simulink model "Test"  (R2022a)
settings: Solver=VariableStepAuto  StartTime=0.0  StopTime=10  RelTol=1e-3
values from neighbouring files (symbols this model uses):
  kd_altitude = 0.475    [QuadcopterParameters.m]
  kd_attitude = 40    [QuadcopterParameters.m]
  KD_position = 0.85    [QuadcopterParameters.m]
  ki_altitude = 0.0275    [QuadcopterParameters.m]
  ki_attitude = 5    [QuadcopterParameters.m]
  KP_altitude = 0.15    [QuadcopterParameters.m]
  kp_attitude = 8.5    [QuadcopterParameters.m]
  KP_position = 0.175    [QuadcopterParameters.m]
  planeX = 30    [QuadcopterParameters.m]
  planeY = 30    [QuadcopterParameters.m]
  planeZ = 0.2    [QuadcopterParameters.m]
  propHoverSpeed = 600    [QuadcopterParameters.m]
  target = wayPoints(:,end)    [QuadcopterParameters.m]
  timeStamp = zeros(length(xWaypt),1)    [QuadcopterParameters.m]
  wayPoints = [xWaypt yWaypt zWaypt]'    [QuadcopterParameters.m]
  xrot = 0    [QuadcopterParameters.m]
  xStart = 0    [QuadcopterParameters.m]
  yrot = 0    [QuadcopterParameters.m]
  yStart = 0    [QuadcopterParameters.m]
  zrot = 0    [QuadcopterParameters.m]
  zStart = 0.06    [QuadcopterParameters.m]
undefined symbols (not defined in the file or in its folder): X, Y, Z
libraries: sm_lib x88, fl_lib x44, nesl_utility x37, slpidlib x4
(part 1 of 4)
settings Model: Creator=ADMIN  LastModifiedBy=ADMIN

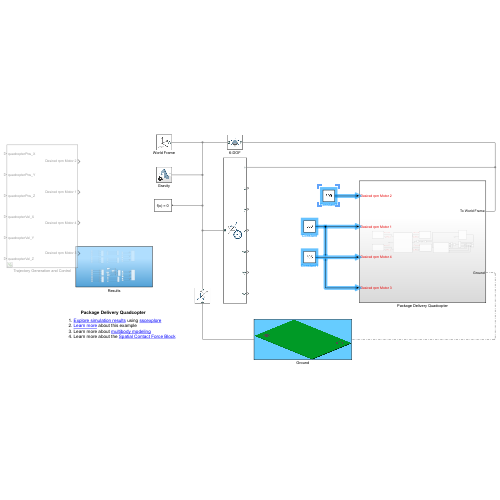
[thumbnail: Simulink's stored preview of the top-level diagram]
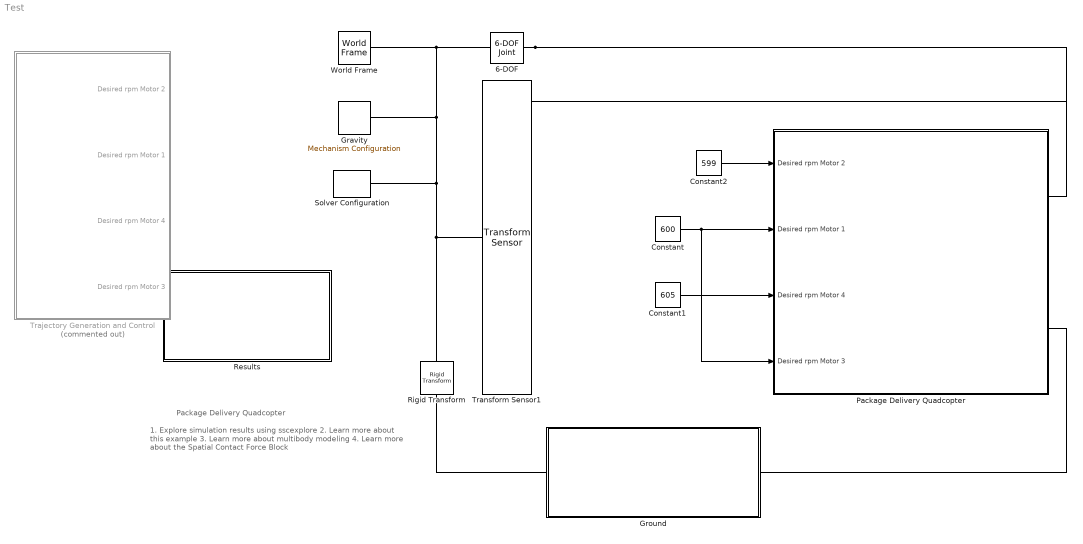
== system Test ==
  note: 1. Explore simulation results using sscexplore
      | 2. Learn more about this example
      | 3. Learn more about multibody modeling
      | 4. Learn more about the Spatial Contact Force Block
  note: Package Delivery Quadcopter
  6-DOF : sm_lib/Joints/6-DOF Joint  JointMode=Normal  SenseConstraintForce=off  SenseConstraintForceX=off  SenseConstraintForceY=off  SenseConstraintForceZ=off  SenseConstraintTorque=off  SenseConstraintTorqueX=off  SenseConstraintTorqueY=off  SenseConstraintTorqueZ=off  SenseTotalForce=off  SenseTotalForceX=off  SenseTotalForceY=off  SenseTotalForceZ=off  SenseTotalTorque=off  SenseTotalTorqueX=off  SenseTotalTorqueY=off  SenseTotalTorqueZ=off  CompositeWrenchDir=FollowerOnBase  CompositeWrenchFrame=BaseFrame  PxEquilibriumPosition=0  PxEquilibriumPositionUnits=m  PxSpringStiffness=0  PxSpringStiffnessUnits=N/m  PxDampingCoefficient=0  PxDampingCoefficientUnits=N/(m/s)  PxTorqueActuationMode=NoTorque  PxMotionActuationMode=ComputedMotion  PxSensePosition=off  PxSenseVelocity=off  PxSenseAcceleration=off  PxSenseTorqueForce=off  PxSenseLowerLimitTorqueForce=off  PxSenseUpperLimitTorqueForce=off  PxLowerLimitSpecify=off  PxLowerLimitBound=-1  PxLowerLimitBoundUnits=m  PxLowerLimitStiffness=1e6  PxLowerLimitStiffnessUnits=N/m  PxLowerLimitDamping=1e3  PxLowerLimitDampingUnits=N/(m/s)  PxLowerLimitTransitionRegionWidth=1e-4  PxLowerLimitTransitionRegionWidthUnits=m  PxUpperLimitSpecify=off  PxUpperLimitBound=1  PxUpperLimitBoundUnits=m  PxUpperLimitStiffness=1e6  PxUpperLimitStiffnessUnits=N/m  PxUpperLimitDamping=1e3  PxUpperLimitDampingUnits=N/(m/s)  PxUpperLimitTransitionRegionWidth=1e-4  PxUpperLimitTransitionRegionWidthUnits=m  PxPositionTargetSpecify=on  PxPositionTargetPriority=High  PxPositionTargetValue=xStart  PxPositionTargetValueUnits=m  PxVelocityTargetSpecify=off  PxVelocityTargetPriority=High  PxVelocityTargetValue=0  PxVelocityTargetValueUnits=m/s  PyEquilibriumPosition=0  PyEquilibriumPositionUnits=m  PySpringStiffness=0  PySpringStiffnessUnits=N/m  PyDampingCoefficient=0  PyDampingCoefficientUnits=N/(m/s)  PyTorqueActuationMode=NoTorque  PyMotionActuationMode=ComputedMotion  PySensePosition=off  PySenseVelocity=off  PySenseAcceleration=off  PySenseTorqueForce=off  PySenseLowerLimitTorqueForce=off  PySenseUpperLimitTorqueForce=off  PyLowerLimitSpecify=off  PyLowerLimitBound=-1  PyLowerLimitBoundUnits=m  PyLowerLimitStiffness=1e6  PyLowerLimitStiffnessUnits=N/m  PyLowerLimitDamping=1e3  PyLowerLimitDampingUnits=N/(m/s)  PyLowerLimitTransitionRegionWidth=1e-4  PyLowerLimitTransitionRegionWidthUnits=m  PyUpperLimitSpecify=off  PyUpperLimitBound=1  PyUpperLimitBoundUnits=m  PyUpperLimitStiffness=1e6  PyUpperLimitStiffnessUnits=N/m  PyUpperLimitDamping=1e3  PyUpperLimitDampingUnits=N/(m/s)  PyUpperLimitTransitionRegionWidth=1e-4  PyUpperLimitTransitionRegionWidthUnits=m  PyPositionTargetSpecify=on  PyPositionTargetPriority=High  PyPositionTargetValue=yStart  PyPositionTargetValueUnits=m  PyVelocityTargetSpecify=off  PyVelocityTargetPriority=High  PyVelocityTargetValue=0  PyVelocityTargetValueUnits=m/s  PzEquilibriumPosition=0  PzEquilibriumPositionUnits=m  PzSpringStiffness=0  PzSpringStiffnessUnits=N/m  PzDampingCoefficient=0  PzDampingCoefficientUnits=N/(m/s)  PzTorqueActuationMode=NoTorque  PzMotionActuationMode=ComputedMotion  PzSensePosition=off  PzSenseVelocity=off  PzSenseAcceleration=off  PzSenseTorqueForce=off  PzSenseLowerLimitTorqueForce=off  PzSenseUpperLimitTorqueForce=off  PzLowerLimitSpecify=off  PzLowerLimitBound=-1  PzLowerLimitBoundUnits=m  PzLowerLimitStiffness=1e6  PzLowerLimitStiffnessUnits=N/m  PzLowerLimitDamping=1e3  PzLowerLimitDampingUnits=N/(m/s)  PzLowerLimitTransitionRegionWidth=1e-4  PzLowerLimitTransitionRegionWidthUnits=m  PzUpperLimitSpecify=off  PzUpperLimitBound=1  PzUpperLimitBoundUnits=m  PzUpperLimitStiffness=1e6  PzUpperLimitStiffnessUnits=N/m  PzUpperLimitDamping=1e3  PzUpperLimitDampingUnits=N/(m/s)  PzUpperLimitTransitionRegionWidth=1e-4  PzUpperLimitTransitionRegionWidthUnits=m  PzPositionTargetSpecify=on  PzPositionTargetPriority=High  PzPositionTargetValue=zStart  PzPositionTargetValueUnits=m  PzVelocityTargetSpecify=off  PzVelocityTargetPriority=High  PzVelocityTargetValue=0  PzVelocityTargetValueUnits=m/s  SphDefPosRotationMethod=None  SphDefPosRotationAngleUnits=deg  SphDefPosRotationStandardAxis=+Z  SphDefPosRotationAngle=0.0  SphDefPosRotationArbitraryAxis=[0 0 1]  SphDefPosFollAlignAxisA=+X  SphDefPosBaseAlignAxisA=+Y  SphDefPosFollAlignAxisB=+Y  SphDefPosBaseAlignAxisB=+Z  SphDefPosRotationSequenceAxes=FollowerAxes  SphDefPosRotationSequence=XYX  SphDefPosRotationSequenceAngles=[0 0 0]  SphDefPosRotationSequenceAnglesUnits=deg  SphDefPosRotationMatrix=[1 0 0; 0 1 0; 0 0 1]  SphEqPosRotationMethod=None  SphEqPosRotationAngleUnits=deg  SphEqPosRotationStandardAxis=+Z  SphEqPosRotationAngle=0.0  SphEqPosRotationArbitraryAxis=[0 0 1]  SphEqPosFollAlignAxisA=+X  SphEqPosBaseAlignAxisA=+Y  SphEqPosFollAlignAxisB=+Y  SphEqPosBaseAlignAxisB=+Z  SphEqPosRotationSequenceAxes=FollowerAxes  SphEqPosRotationSequence=XYX  SphEqPosRotationSequenceAngles=[0 0 0]  SphEqPosRotationSequenceAnglesUnits=deg  SphEqPosRotationMatrix=[1 0 0; 0 1 0; 0 0 1]  SphSpringStiffness=0  SphSpringStiffnessUnits=N*m/deg  SphDampingCoefficient=0  SphDampingCoefficientUnits=N*m/(deg/s)  SphActuateTorqueX=off  SphActuateTorqueY=off  SphActuateTorqueZ=off  SphActuateTorque=off  SphTorqueActuationMode=NoTorque  SphMotionActuationMode=ComputedMotion  SphActuationFrame=BaseFrame  SphSensePosition=off  SphSenseVelocityX=off  SphSenseVelocityY=off  SphSenseVelocityZ=off  SphSenseVelocity=off  SphSenseAccelerationX=off  SphSenseAccelerationY=off  SphSenseAccelerationZ=off  SphSenseAcceleration=off  SphSenseTorqueX=off  SphSenseTorqueY=off  SphSenseTorqueZ=off  SphSenseTorqueForce=off  SphSenseLowerLimitTorqueMag=off  SphSenseUpperLimitTorqueMag=off  SphSensingFrame=BaseFrame  SphLowerLimitSpecify=off  SphLowerLimitBound=15  SphLowerLimitBoundUnits=deg  SphLowerLimitStiffness=1e4  SphLowerLimitStiffnessUnits=N*m/deg  SphLowerLimitDamping=10  SphLowerLimitDampingUnits=N*m/(deg/s)  SphLowerLimitTransitionRegionWidth=0.1  SphLowerLimitTransitionRegionWidthUnits=deg  SphUpperLimitSpecify=off  SphUpperLimitBound=45  SphUpperLimitBoundUnits=deg  SphUpperLimitStiffness=1e4  SphUpperLimitStiffnessUnits=N*m/deg  SphUpperLimitDamping=10  SphUpperLimitDampingUnits=N*m/(deg/s)  SphUpperLimitTransitionRegionWidth=0.1  SphUpperLimitTransitionRegionWidthUnits=deg  SphPositionTargetRotationMethod=RotationSequence  SphPositionTargetRotationAngleUnits=deg  SphPositionTargetRotationStandardAxis=+Y  SphPositionTargetRotationAngle=0  SphPositionTargetRotationArbitraryAxis=[0 0 1]  SphPositionTargetFollAlignAxisA=+X  SphPositionTargetBaseAlignAxisA=+Y  SphPositionTargetFollAlignAxisB=+Y  SphPositionTargetBaseAlignAxisB=+Z  SphPositionTargetRotationSequenceAxes=FollowerAxes  SphPositionTargetRotationSequence=XYZ  SphPositionTargetRotationSequenceAngles=[xrot yrot zrot]  SphPositionTargetRotationSequenceAnglesUnits=deg  SphPositionTargetRotationMatrix=[1 0 0; 0 1 0; 0 0 1]  SphPositionTargetSpecify=on  SphPositionTargetPriority=High  SphVelocityTargetValue=[0 0 0]  SphVelocityTargetValueUnits=deg/s  SphVelocityTargetSpecify=off  SphVelocityTargetPriority=High  SphVelocityTargetInFollowerFrame=on
  Constant : Constant  Value=600
  Constant1 : Constant  Value=605
  Constant2 : Constant  Value=599
  Gravity : sm_lib/Utilities/Mechanism Configuration  UniformGravity=Constant  GravityVector=[0 0 -9.80665]  GravityUnits=m/s^2  LinearizationDelta=0.001  JointModeTransitionNonlinearIterations=2
  Ground : Subsystem
      mask Display:
      | image(fullfile(matlabroot,'toolbox','physmod','sm','smdemos',...
      |     'quadcopter_package_delivery','images','ground.PNG'));
  Package Delivery Quadcopter : Subsystem
  "Results " : Subsystem
  Rigid Transform : sm_lib/Frames and Transforms/Rigid Transform  TranslationMethod=StandardAxis  TranslationStandardOffset=0.25  TranslationLengthUnit=m  TranslationStandardAxis=-Z  TranslationCartesianOffset=[0 0 0]  TranslationROffset=0  TranslationROffsetUnits=m  TranslationZOffset=0  TranslationZOffsetUnits=m  TranslationThetaOffset=0  TranslationThetaOffsetUnits=deg  RotationMethod=None  RotationAngleUnits=deg  RotationStandardAxis=+Z  RotationAngle=0.0  RotationArbitraryAxis=[0 0 1]  FollAlignAxisA=+X  BaseAlignAxisA=+Y  FollAlignAxisB=+Y  BaseAlignAxisB=+Z  RotationSequenceAxes=FollowerAxes  RotationSequence=XYX  RotationSequenceAngles=[0 0 0]  RotationSequenceAnglesUnits=deg  RotationMatrix=[1 0 0; 0 1 0; 0 0 1]
  Solver Configuration : nesl_utility/Solver Configuration  PhysicalDomain=network_engine_domain  SubClassName=solver  LeftPortType=input  RightPortType=generic  Tones=[]  Harmonics=[]  SimulateNoise=off  Profile=off  UseLocalSampling=off  EnableSwitchedLinearOptims=on  FrequencyDomain=off  UseCCode=off  RelTol=0.001  AbsTol=1e-06  MinStep=1e-09  ToWorkspace=off  RevertToSquareIcSolve=off  NumHomotopyIterations=100  PhasorMode=off  PhasorModeNumHarmonics=1  IndexReductionMethod=DerivativeReplacement  DoDC=off  ResidualTolerance=1e-09  UseLocalSolver=off  LocalSolverChoice=NE_BACKWARD_EULER_ADVANCER  LocalSolverSampleTime=Ts  DoFixedCost=off  MaxNonlinIter=3  MaxModeIter=2  ComputeImpulses=off  ImpulseIterations=2  LinearAlgebra=auto  LinearAlgebraNumThread=0  EquationFormulation=NE_TIME_EF  DelaysMemoryBudget=1024  AutomaticFiltering=on  FilteringTimeConstant=0.001  PartitionStorageMethod=AS_NEEDED  PartitionMemoryBudget=1024  PartitionMethod=ROBUST
      settings: SourceProductBaseCode=SS,PW,VE
  Trajectory Generation and Control : Subsystem  Commented=on
  Transform Sensor1 : sm_lib/Frames and Transforms/Transform Sensor  MeasurementFrame=NonRotatingBase  SenseAngle=off  SenseAxis=off  SenseAngle1=off  SenseAngle2=off  SenseAngle3=off  SenseQ=off  SenseR=off  SenseOmegaX=off  SenseOmegaY=off  SenseOmegaZ=off  SenseOmega1=off  SenseOmega2=off  SenseOmega3=off  SenseQDot=off  SenseRDot=off  SenseAlphaX=off  SenseAlphaY=off  SenseAlphaZ=off  SenseAlpha1=off  SenseAlpha2=off  SenseAlpha3=off  SenseQDDot=off  SenseRDDot=off  SenseX=on  SenseY=on  SenseZ=on  SenseRad=off  SenseAzim=off  SenseDist=off  SenseInc=off  SenseXDot=on  SenseYDot=on  SenseZDot=on  SenseRadDot=off  SenseAzimDot=off  SenseDistDot=off  SenseIncDot=off  SenseXDDot=off  SenseYDDot=off  SenseZDDot=off  SenseRadDDot=off  SenseAzimDDot=off  SenseDistDDot=off  SenseIncDDot=off
  World Frame : sm_lib/Frames and Transforms/World Frame
  wires:
  Constant2/1 -> Package Delivery Quadcopter/1(Desired rpm Motor 2)
  Constant1/1 -> Package Delivery Quadcopter/3(Desired rpm Motor 4)
  Constant/1 -> Package Delivery Quadcopter/4(Desired rpm Motor 3), Package Delivery Quadcopter/2("Desired rpm Motor 1 ")
  connections:
  Rigid Transform/LConn1 -- Transform Sensor1/LConn1 -- Gravity/RConn1 -- 6-DOF/LConn1 -- World Frame/RConn1 -- Solver Configuration/RConn1
  6-DOF/RConn1 -- Transform Sensor1/RConn1 -- Package Delivery Quadcopter/RConn1
  Package Delivery Quadcopter/RConn2 -- Ground/LConn1
  Rigid Transform/RConn1 -- Ground/RConn1

== system Test/Ground ==
  Ground : sm_lib/Body Elements/Brick Solid  GraphicAmbientColor=[0.15 0.15 0.15 1.0]  BasedOnType=Density  BrickDimensions=[planeX planeY planeZ]  BrickDimensionUnits=m  CenterOfMass=[0 0 0]  CenterOfMassUnits=m  GraphicDiffuseColor=[0.0 0.8 0.2]  Density=1000  DensityUnits=kg/m^3  DoExposeReferenceFrame=on  GraphicEmissiveColor=[0.0 0.0 0.0 1.0]  ExportEntireGeometry=on  SerializedFrames=<Frames><Frame><Id>Frame1</Id><Value><Name>Lp</Name><Origin><Source>GeometricFeature</Source><FeatureName>+z surface</FeatureName></Origin><PrimaryAxis><DefinedDirection>+Z</DefinedDirection><Source>ReferenceFrame</Source><SourceDirection>+Z</SourceDirection><FeatureName></FeatureName></PrimaryAxis><SecondaryAxis><DefinedDirection>+X</DefinedDirection><Source>ReferenceFrame</Source><SourceDirection>+X</SourceDirection><FeatureName></FeatureName></SecondaryAxis></Value></Frame></Frames>  MarkerShape=Sphere  MarkerSize=10  GraphicType=FromGeometry  InertiaType=CalculateFromGeometry  Mass=1  MassUnits=kg  MomentsOfInertia=[1 1 1]  MomentsOfInertiaUnits=kg*m^2  GraphicOpacity=1  ProductsOfInertia=[0 0 0]  ProductsOfInertiaUnits=kg*m^2  GraphicShininess=75  GraphicSpecularColor=[0.5 0.5 0.5 1.0]  GraphicVisPropType=SimpleVisualProperties
  Launchpad : sm_lib/Body Elements/Extruded Solid  GraphicAmbientColor=[0.15 0.15 0.15 1.0]  BasedOnType=Density  CenterOfMass=[0 0 0]  CenterOfMassUnits=m  GraphicDiffuseColor=[0.4 0.4 0.4]  ExportConvexHullGeometry=off  ExtrusionCrossSection=[0.15 0.15; -0.15 0.15; -0.15 0.75; -0.6 0.75; -0.6 -0.75; -0.15 -0.75; -0.15 -0.15; 0.15 -0.15; 0.15 -0.75; 0.6 -0.75; 0.6 0.75; 0.15 0.75]*0.25  ExtrusionCrossSectionUnits=m  Density=1  DensityUnits=kg/m^3  DoExposeReferenceFrame=on  GraphicEmissiveColor=[0.0 0.0 0.0 1.0]  ExportEntireGeometry=off  ExtrusionLength=0.002  ExtrusionLengthUnits=m  ExtrusionType=General  SerializedFrames=<Frames/>  MarkerShape=Sphere  MarkerSize=10  GraphicType=FromGeometry  InertiaType=CalculateFromGeometry  Mass=1  MassUnits=kg  MomentsOfInertia=[1 1 1]  MomentsOfInertiaUnits=kg*m^2  PolygonNumSides=3  GraphicOpacity=1.0  PolygonOuterRadius=1  PolygonOuterRadiusUnits=m  ProductsOfInertia=[0 0 0]  ProductsOfInertiaUnits=kg*m^2  GraphicShininess=75  GraphicSpecularColor=[0.5 0.5 0.5 1.0]  GraphicVisPropType=SimpleVisualProperties
  Revolved Solid : sm_lib/Body Elements/Revolved Solid  GraphicAmbientColor=[0.15 0.15 0.15 1.0]  BasedOnType=Density  CenterOfMass=[0 0 0]  CenterOfMassUnits=m  GraphicDiffuseColor=[0.4 0.4 0.4]  ExportConvexHullGeometry=off  Density=1000  DensityUnits=kg/m^3  DoExposeReferenceFrame=on  GraphicEmissiveColor=[0.0 0.0 0.0 1.0]  ExportEntireGeometry=off  SerializedFrames=<Frames/>  MarkerShape=Sphere  MarkerSize=10  GraphicType=FromGeometry  InertiaType=CalculateFromGeometry  Mass=1  MassUnits=kg  MomentsOfInertia=[1 1 1]  MomentsOfInertiaUnits=kg*m^2  GraphicOpacity=1.0  ProductsOfInertia=[0 0 0]  ProductsOfInertiaUnits=kg*m^2  RevolutionCrossSection=[0.5 0.001; 0.5 -0.001; 0.75 -0.001; 0.75 0.001]*0.65  RevolutionCrossSectionUnits=m  RevolutionAngle=180  RevolutionAngleUnits=deg  RevolutionExtent=Full  GraphicShininess=75  GraphicSpecularColor=[0.5 0.5 0.5 1.0]  GraphicVisPropType=SimpleVisualProperties
  Rigid Transform1 : sm_lib/Frames and Transforms/Rigid Transform  TranslationMethod=Cartesian  TranslationStandardOffset=0  TranslationLengthUnit=m  TranslationStandardAxis=+Z  TranslationCartesianOffset=[xStart yStart 0 ]  TranslationROffset=0  TranslationROffsetUnits=m  TranslationZOffset=0  TranslationZOffsetUnits=m  TranslationThetaOffset=0  TranslationThetaOffsetUnits=deg  RotationMethod=None  RotationAngleUnits=deg  RotationStandardAxis=+Z  RotationAngle=0.0  RotationArbitraryAxis=[0 0 1]  FollAlignAxisA=+X  BaseAlignAxisA=+Y  FollAlignAxisB=+Y  BaseAlignAxisB=+Z  RotationSequenceAxes=FollowerAxes  RotationSequence=XYX  RotationSequenceAngles=[0 0 0]  RotationSequenceAnglesUnits=deg  RotationMatrix=[1 0 0; 0 1 0; 0 0 1]
  Rigid Transform12 : sm_lib/Frames and Transforms/Rigid Transform  TranslationMethod=Cartesian  TranslationStandardOffset=0  TranslationLengthUnit=m  TranslationStandardAxis=+Z  TranslationCartesianOffset=[target(1) target(2) 0 ]  TranslationROffset=0  TranslationROffsetUnits=m  TranslationZOffset=0  TranslationZOffsetUnits=m  TranslationThetaOffset=0  TranslationThetaOffsetUnits=deg  RotationMethod=None  RotationAngleUnits=deg  RotationStandardAxis=+Z  RotationAngle=0.0  RotationArbitraryAxis=[0 0 1]  FollAlignAxisA=+X  BaseAlignAxisA=+Y  FollAlignAxisB=+Y  BaseAlignAxisB=+Z  RotationSequenceAxes=FollowerAxes  RotationSequence=XYX  RotationSequenceAngles=[0 0 0]  RotationSequenceAnglesUnits=deg  RotationMatrix=[1 0 0; 0 1 0; 0 0 1]
  Target Marker : sm_lib/Body Elements/Revolved Solid  GraphicAmbientColor=[0.15 0.15 0.15 1.0]  BasedOnType=Density  CenterOfMass=[0 0 0]  CenterOfMassUnits=m  GraphicDiffuseColor=[0.4 0.4 0.4]  ExportConvexHullGeometry=off  Density=1000  DensityUnits=kg/m^3  DoExposeReferenceFrame=on  GraphicEmissiveColor=[0.0 0.0 0.0 1.0]  ExportEntireGeometry=off  SerializedFrames=<Frames/>  MarkerShape=Sphere  MarkerSize=10  GraphicType=FromGeometry  InertiaType=CalculateFromGeometry  Mass=1  MassUnits=kg  MomentsOfInertia=[1 1 1]  MomentsOfInertiaUnits=kg*m^2  GraphicOpacity=1.0  ProductsOfInertia=[0 0 0]  ProductsOfInertiaUnits=kg*m^2  RevolutionCrossSection=[0.5 0.001; 0.5 -0.001; 0.75 -0.001; 0.75 0.001]*0.75  RevolutionCrossSectionUnits=m  RevolutionAngle=180  RevolutionAngleUnits=deg  RevolutionExtent=Full  GraphicShininess=75  GraphicSpecularColor=[0.5 0.5 0.5 1.0]  GraphicVisPropType=SimpleVisualProperties
  Package : PMIOPort  Side=Left
  World Frame : PMIOPort  Port=2  Side=Right
  connections:
  Package/RConn1 -- Ground/LConn2
  Rigid Transform12/RConn1 -- Target Marker/RConn1
  Rigid Transform12/LConn1 -- Rigid Transform1/LConn1 -- Ground/LConn1
  Launchpad/RConn1 -- Revolved Solid/RConn1 -- Rigid Transform1/RConn1
  World Frame/RConn1 -- Ground/RConn1

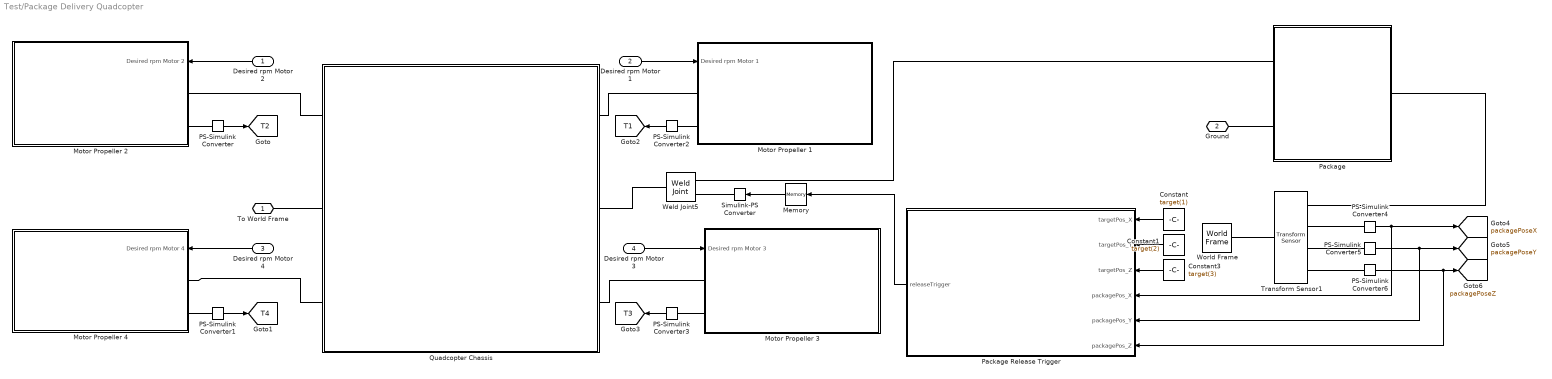
== system Test/Package Delivery Quadcopter ==
  Desired rpm Motor 2 : Inport
  "Desired rpm Motor 1 " : Inport  Port=2
  Desired rpm Motor 4 : Inport  Port=3
  Desired rpm Motor 3 : Inport  Port=4
  Constant : Constant  Value=target(1)
  Constant1 : Constant  Value=target(2)
  Constant3 : Constant  Value=target(3)
  Memory : Memory
  Motor Propeller 1 : Subsystem
  Motor Propeller 2 : Subsystem
      mask Display:
      | image(fullfile(matlabroot,'toolbox','physmod','sm','smdemos',...
      |     'quadcopter_package_delivery','images','propeller2.PNG'));
  "Motor Propeller 3 " : Subsystem
      mask Display:
      | image(fullfile(matlabroot,'toolbox','physmod','sm','smdemos',...
      |     'quadcopter_package_delivery','images','propeller3.PNG'));
  Motor Propeller 4 : Subsystem
      mask Display:
      | image(fullfile(matlabroot,'toolbox','physmod','sm','smdemos',...
      |     'quadcopter_package_delivery','images','propeller4.PNG'));
  PS-Simulink Converter{,1..6} (7 alike) : nesl_utility/PS-Simulink Converter  PhysicalDomain=network_engine_domain  SubClassName=ps_output  LeftPortType=input  RightPortType=output  PseudoPeriodic=off  Frequencies=[]  VectorFormat=1-D array  Unit=inherit  AffineConversion=off
      settings: SourceProductBaseCode=SS,PW,VE
  Package : Subsystem
      mask Display:
      | image(fullfile(matlabroot,'toolbox','physmod','sm','smdemos',...
      |     'quadcopter_package_delivery','images','medical_kit.png'));
  Package Release Trigger : MATLAB Function  TreatAsAtomicUnit=on
  Quadcopter Chassis : Subsystem
  Simulink-PS Converter : nesl_utility/Simulink-PS Converter  PhysicalDomain=network_engine_domain  SubClassName=ps_input  LeftPortType=input  RightPortType=output  PseudoPeriodic=off  Frequencies=[]  NoiseDistribution=none  NoiseParameters=[]  Unit=1  AffineConversion=off  FilteringAndDerivatives=provide  SimscapeFilterOrder=1  InputFilterTimeConstant=0.001  UdotUserProvided=0
      settings: SourceProductBaseCode=SS,PW,VE
  Transform Sensor1 : sm_lib/Frames and Transforms/Transform Sensor  MeasurementFrame=World  SenseAngle=off  SenseAxis=off  SenseAngle1=off  SenseAngle2=off  SenseAngle3=off  SenseQ=off  SenseR=off  SenseOmegaX=off  SenseOmegaY=off  SenseOmegaZ=off  SenseOmega1=off  SenseOmega2=off  SenseOmega3=off  SenseQDot=off  SenseRDot=off  SenseAlphaX=off  SenseAlphaY=off  SenseAlphaZ=off  SenseAlpha1=off  SenseAlpha2=off  SenseAlpha3=off  SenseQDDot=off  SenseRDDot=off  SenseX=on  SenseY=on  SenseZ=on  SenseRad=off  SenseAzim=off  SenseDist=off  SenseInc=off  SenseXDot=off  SenseYDot=off  SenseZDot=off  SenseRadDot=off  SenseAzimDot=off  SenseDistDot=off  SenseIncDot=off  SenseXDDot=off  SenseYDDot=off  SenseZDDot=off  SenseRadDDot=off  SenseAzimDDot=off  SenseDistDDot=off  SenseIncDDot=off
  Weld Joint5 : sm_lib/Joints/Weld Joint  JointMode=ProvidedByInput  SenseConstraintForce=off  SenseConstraintForceX=off  SenseConstraintForceY=off  SenseConstraintForceZ=off  SenseConstraintTorque=off  SenseConstraintTorqueX=off  SenseConstraintTorqueY=off  SenseConstraintTorqueZ=off  SenseTotalForce=off  SenseTotalForceX=off  SenseTotalForceY=off  SenseTotalForceZ=off  SenseTotalTorque=off  SenseTotalTorqueX=off  SenseTotalTorqueY=off  SenseTotalTorqueZ=off  CompositeWrenchDir=FollowerOnBase  CompositeWrenchFrame=BaseFrame
  World Frame : sm_lib/Frames and Transforms/World Frame
  To World Frame : PMIOPort  Side=Right
  Ground : PMIOPort  Port=2  Side=Right
  tag scope: T1=global, T2=global, T3=global, T4=global, packagePoseX=global, packagePoseY=global, packagePoseZ=global
  wires:
  PS-Simulink Converter/1 -> [T2]
  PS-Simulink Converter1/1 -> [T4]
  PS-Simulink Converter2/1 -> [T1]
  PS-Simulink Converter3/1 -> [T3]
  Desired rpm Motor 2/1 -> Motor Propeller 2/1(Desired rpm Motor 2)
  "Desired rpm Motor 1 "/1 -> Motor Propeller 1/1(Desired rpm Motor 1)
  Desired rpm Motor 4/1 -> Motor Propeller 4/1(Desired rpm Motor 4)
  Desired rpm Motor 3/1 -> "Motor Propeller 3 "/1(Desired rpm Motor 3)
  Memory/1 -> Simulink-PS Converter/1
  PS-Simulink Converter4/1 -> Package Release Trigger/4(packagePos_X), [packagePoseX]
  PS-Simulink Converter6/1 -> Package Release Trigger/6(packagePos_Z), [packagePoseZ]
  Package Release Trigger/1(releaseTrigger) -> Memory/1
  PS-Simulink Converter5/1 -> Package Release Trigger/5(packagePos_Y), [packagePoseY]
  Constant/1 -> Package Release Trigger/1(targetPos_X)
  Constant1/1 -> Package Release Trigger/2(targetPos_Y)
  Constant3/1 -> Package Release Trigger/3(targetPos_Z)
  connections:
  Motor Propeller 2/LConn1 -- Quadcopter Chassis/LConn1
  Motor Propeller 1/LConn1 -- Quadcopter Chassis/RConn1
  PS-Simulink Converter/LConn1 -- Motor Propeller 2/LConn2
  PS-Simulink Converter1/LConn1 -- Motor Propeller 4/LConn2
  PS-Simulink Converter2/LConn1 -- Motor Propeller 1/LConn2
  PS-Simulink Converter3/LConn1 -- "Motor Propeller 3 "/LConn2
  "Motor Propeller 3 "/LConn1 -- Quadcopter Chassis/RConn3
  Transform Sensor1/RConn1 -- Package/RConn1
  Ground/RConn1 -- Package/LConn2
  Transform Sensor1/RConn4 -- PS-Simulink Converter6/LConn1
  Transform Sensor1/RConn2 -- PS-Simulink Converter4/LConn1
  Transform Sensor1/RConn3 -- PS-Simulink Converter5/LConn1
  Simulink-PS Converter/RConn1 -- Weld Joint5/LConn2
  Package/LConn1 -- Weld Joint5/LConn1
  World Frame/RConn1 -- Transform Sensor1/LConn1
  Motor Propeller 4/LConn1 -- Quadcopter Chassis/LConn3
  To World Frame/RConn1 -- Quadcopter Chassis/LConn2
  Quadcopter Chassis/RConn2 -- Weld Joint5/RConn1

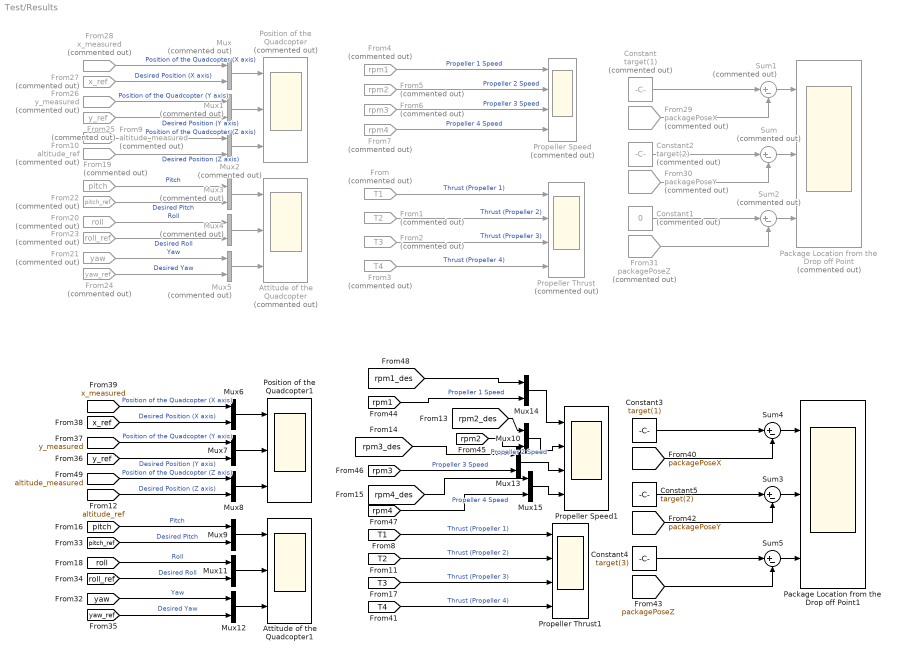
== system Test/Results  ==
  Attitude of the Quadcopter : Scope  Commented=on  NumInputPorts=3
  Attitude of the Quadcopter1 : Scope  NumInputPorts=3
  Constant : Constant  Commented=on  Value=target(1)
  Constant1 : Constant  Commented=on  Value=0
  Constant2 : Constant  Commented=on  Value=target(2)
  Constant3 : Constant  Value=target(1)
  Constant4 : Constant  Value=target(3)
  Constant5 : Constant  Value=target(2)
  From : From  Commented=on  GotoTag=T1  TagVisibility=global
  From1 : From  Commented=on  GotoTag=T2  TagVisibility=global
  From10 : From  Commented=on  GotoTag=altitude_ref  TagVisibility=global
  From19 : From  Commented=on  GotoTag=pitch  TagVisibility=global
  From2 : From  Commented=on  GotoTag=T3  TagVisibility=global
  From20 : From  Commented=on  GotoTag=roll  TagVisibility=global
  From21 : From  Commented=on  GotoTag=yaw  TagVisibility=global
  From22 : From  Commented=on  GotoTag=pitch_ref  TagVisibility=global
  From23 : From  Commented=on  GotoTag=roll_ref  TagVisibility=global
  From24 : From  Commented=on  GotoTag=yaw_ref  TagVisibility=global
  From25 : From  Commented=on  GotoTag=y_ref  TagVisibility=global
  From26 : From  Commented=on  GotoTag=y_measured  TagVisibility=global
  From27 : From  Commented=on  GotoTag=x_ref  TagVisibility=global
  From28 : From  Commented=on  GotoTag=x_measured  TagVisibility=global
  From29 : From  Commented=on  GotoTag=packagePoseX  TagVisibility=global
  From3 : From  Commented=on  GotoTag=T4  TagVisibility=global
  From30 : From  Commented=on  GotoTag=packagePoseY  TagVisibility=global
  From31 : From  Commented=on  GotoTag=packagePoseZ  TagVisibility=global
  From4 : From  Commented=on  GotoTag=rpm1  TagVisibility=global
  From5 : From  Commented=on  GotoTag=rpm2  TagVisibility=global
  From6 : From  Commented=on  GotoTag=rpm3  TagVisibility=global
  From7 : From  Commented=on  GotoTag=rpm4  TagVisibility=global
  From9 : From  Commented=on  GotoTag=altitude_measured  TagVisibility=global
  Mux{,1..5} (6 alike) : Mux  Commented=on  Inputs=2
  Mux{6..15} (10 alike) : Mux  Inputs=2
  Package Location from the Drop off Point : Scope  Commented=on  NumInputPorts=3
  Package Location from the Drop off Point1 : Scope  NumInputPorts=3
  Position of the Quadcopter : Scope  Commented=on  NumInputPorts=3
  Position of the Quadcopter1 : Scope  NumInputPorts=3
  Propeller Speed : Scope  Commented=on  NumInputPorts=4
  Propeller Speed1 : Scope  NumInputPorts=4
  Propeller Thrust : Scope  Commented=on  NumInputPorts=4
  Propeller Thrust1 : Scope  NumInputPorts=4
  Sum : Sum  Commented=on  Inputs=|+-
  Sum1 : Sum  Commented=on  Inputs=|+-
  Sum2 : Sum  Commented=on  Inputs=|+-
  Sum3 : Sum  Inputs=|+-
  Sum4 : Sum  Inputs=|+-
  Sum5 : Sum  Inputs=|+-
  wires:
  From4/1 -> Propeller Speed/1  "Propeller 1 Speed"
  From5/1 -> Propeller Speed/2  "Propeller 2 Speed"
  From6/1 -> Propeller Speed/3  "Propeller 3 Speed"
  From7/1 -> Propeller Speed/4  "Propeller 4 Speed"
  From10/1 -> Mux2/2  "Desired Position (Z axis)"
  From9/1 -> Mux2/1  "Position of the Quadcopter (Z axis)"
  From19/1 -> Mux3/1  "Pitch"
  From20/1 -> Mux4/1  "Roll"
  From21/1 -> Mux5/1  "Yaw"
  From22/1 -> Mux3/2  "Desired Pitch"
  From23/1 -> Mux4/2  "Desired Roll"
  From24/1 -> Mux5/2  "Desired Yaw"
  From25/1 -> Mux1/2  "Desired Position (Y axis)"
  From26/1 -> Mux1/1  "Position of the Quadcopter (Y axis)"
  From27/1 -> Mux/2  "Desired Position (X axis)"
  From28/1 -> Mux/1  "Position of the Quadcopter (X axis)"
  From31/1 -> Sum2/2
  Constant1/1 -> Sum2/1
  Constant2/1 -> Sum/1
  From30/1 -> Sum/2
  Constant/1 -> Sum1/1
  From29/1 -> Sum1/2
  Sum/1 -> Package Location from the Drop off Point/2
  Sum2/1 -> Package Location from the Drop off Point/3
  Mux1/1 -> Position of the Quadcopter/2
  Mux/1 -> Position of the Quadcopter/1
  Mux2/1 -> Position of the Quadcopter/3
  Mux4/1 -> Attitude of the Quadcopter/2
  Mux3/1 -> Attitude of the Quadcopter/1
  Mux5/1 -> Attitude of the Quadcopter/3
  From2/1 -> Propeller Thrust/3  "Thrust (Propeller 3)"
  From1/1 -> Propeller Thrust/2  "Thrust (Propeller 2)"
  From/1 -> Propeller Thrust/1  "Thrust (Propeller 1)"
  From3/1 -> Propeller Thrust/4  "Thrust (Propeller 4)"
  Sum1/1 -> Package Location from the Drop off Point/1
  [rpm3_des] -> Mux13/1
  [rpm3] -> Mux13/2  "Propeller 3 Speed"
  Mux15/1 -> Propeller Speed1/4
  Mux6/1 -> Position of the Quadcopter1/1
  [T3] -> Propeller Thrust1/3  "Thrust (Propeller 3)"
  Mux10/1 -> Propeller Speed1/2
  Sum4/1 -> Package Location from the Drop off Point1/1
  [T4] -> Propeller Thrust1/4  "Thrust (Propeller 4)"
  Mux12/1 -> Attitude of the Quadcopter1/3
  [pitch_ref] -> Mux9/2  "Desired Pitch"
  Constant3/1 -> Sum4/1
  [yaw] -> Mux12/1  "Yaw"
  [x_ref] -> Mux6/2  "Desired Position (X axis)"
  [rpm2] -> Mux10/2  "Propeller 2 Speed"
  [T2] -> Propeller Thrust1/2  "Thrust (Propeller 2)"
  [x_measured] -> Mux6/1  "Position of the Quadcopter (X axis)"
  Mux9/1 -> Attitude of the Quadcopter1/1
  Mux11/1 -> Attitude of the Quadcopter1/2
  [altitude_ref] -> Mux8/2  "Desired Position (Z axis)"
  Constant5/1 -> Sum3/1
  Sum3/1 -> Package Location from the Drop off Point1/2
  [y_ref] -> Mux7/2  "Desired Position (Y axis)"
  [roll] -> Mux11/1  "Roll"
  [rpm1] -> Mux14/2  "Propeller 1 Speed"
  [y_measured] -> Mux7/1  "Position of the Quadcopter (Y axis)"
  [packagePoseX] -> Sum4/2
  Constant4/1 -> Sum5/1
  [rpm2_des] -> Mux10/1
  [packagePoseZ] -> Sum5/2
  Mux13/1 -> Propeller Speed1/3
  [rpm4] -> Mux15/2  "Propeller 4 Speed"
  [yaw_ref] -> Mux12/2  "Desired Yaw"
  Sum5/1 -> Package Location from the Drop off Point1/3
  [packagePoseY] -> Sum3/2
  Mux14/1 -> Propeller Speed1/1
  [roll_ref] -> Mux11/2  "Desired Roll"
  Mux7/1 -> Position of the Quadcopter1/2
  [rpm1_des] -> Mux14/1
  Mux8/1 -> Position of the Quadcopter1/3
  [pitch] -> Mux9/1  "Pitch"
  [T1] -> Propeller Thrust1/1  "Thrust (Propeller 1)"
  [rpm4_des] -> Mux15/1
  [altitude_measured] -> Mux8/1  "Position of the Quadcopter (Z axis)"

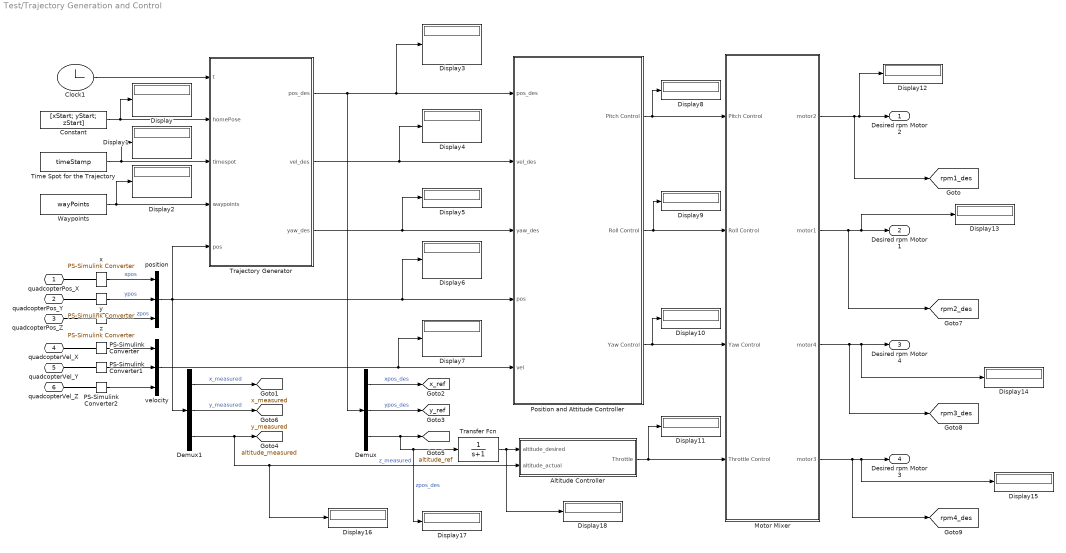
== system Test/Trajectory Generation and Control ==
  Altitude Controller : Subsystem
  Clock1 : Clock
  Constant : Constant  Value=[xStart; yStart; zStart]
  Demux : Demux  Outputs=3
  Demux1 : Demux  Outputs=3
  Display{,1..18} (19 alike) : Display
  Motor Mixer : Subsystem
  PS-Simulink Converter : nesl_utility/PS-Simulink Converter  PhysicalDomain=network_engine_domain  SubClassName=ps_output  LeftPortType=input  RightPortType=output  PseudoPeriodic=off  Frequencies=[]  VectorFormat=1-D array  Unit=inherit  AffineConversion=off
      settings: SourceProductBaseCode=SS,PW,VE
  PS-Simulink Converter1 : nesl_utility/PS-Simulink Converter  PhysicalDomain=network_engine_domain  SubClassName=ps_output  LeftPortType=input  RightPortType=output  PseudoPeriodic=off  Frequencies=[]  VectorFormat=1-D array  Unit=inherit  AffineConversion=off
      settings: SourceProductBaseCode=SS,PW,VE
  PS-Simulink Converter2 : nesl_utility/PS-Simulink Converter  PhysicalDomain=network_engine_domain  SubClassName=ps_output  LeftPortType=input  RightPortType=output  PseudoPeriodic=off  Frequencies=[]  VectorFormat=1-D array  Unit=inherit  AffineConversion=off
      settings: SourceProductBaseCode=SS,PW,VE
  Position and Attitude Controller : Subsystem
  Time Spot for the Trajectory : Constant  Value=timeStamp
  Trajectory Generator : MATLAB Function  TreatAsAtomicUnit=on
  Transfer Fcn : TransferFcn  Denominator=[1 1]
  Waypoints : Constant  Value=wayPoints
  position : Mux  Inputs=3
  velocity : Mux  Inputs=3
  x : nesl_utility/PS-Simulink Converter  PhysicalDomain=network_engine_domain  SubClassName=ps_output  LeftPortType=input  RightPortType=output  PseudoPeriodic=off  Frequencies=[]  VectorFormat=1-D array  Unit=1  AffineConversion=off
      settings: SourceProductBaseCode=SS,PW,VE
  y : nesl_utility/PS-Simulink Converter  PhysicalDomain=network_engine_domain  SubClassName=ps_output  LeftPortType=input  RightPortType=output  PseudoPeriodic=off  Frequencies=[]  VectorFormat=1-D array  Unit=1  AffineConversion=off
      settings: SourceProductBaseCode=SS,PW,VE
  z : nesl_utility/PS-Simulink Converter  PhysicalDomain=network_engine_domain  SubClassName=ps_output  LeftPortType=input  RightPortType=output  PseudoPeriodic=off  Frequencies=[]  VectorFormat=1-D array  Unit=1  AffineConversion=off
      settings: SourceProductBaseCode=SS,PW,VE
  quadcopterPos_X : PMIOPort  Side=Left
  quadcopterPos_Y : PMIOPort  Port=2  Side=Left
  quadcopterPos_Z : PMIOPort  Port=3  Side=Left
  quadcopterVel_X : PMIOPort  Port=4  Side=Left
  quadcopterVel_Y : PMIOPort  Port=5  Side=Left
  quadcopterVel_Z : PMIOPort  Port=6  Side=Left
  Desired rpm Motor 2 : Outport
  Desired rpm Motor 1 : Outport  Port=2
  Desired rpm Motor 4 : Outport  Port=3
  Desired rpm Motor 3 : Outport  Port=4
  tag scope: altitude_measured=global, altitude_ref=global, rpm1_des=global, rpm2_des=global, rpm3_des=global, rpm4_des=global, x_measured=global, x_ref=global, y_measured=global, y_ref=global
  wires:
  z/1 -> position/3  "zpos"
  PS-Simulink Converter1/1 -> velocity/2
  PS-Simulink Converter/1 -> velocity/1
  PS-Simulink Converter2/1 -> velocity/3
  x/1 -> position/1  "xpos"
  position/1 -> Trajectory Generator/5(pos), Demux1/1, Display6/1, Position and Attitude Controller/4(pos)
  Demux/2 -> [y_ref]  "ypos_des"
  Demux/1 -> [x_ref]  "xpos_des"
  Demux/3 -> Display17/1, Transfer Fcn/1, [altitude_ref]  "zpos_des"
  y/1 -> position/2  "ypos"
  Demux1/1 -> [x_measured]  "x_measured"
  Demux1/3 -> [altitude_measured], Altitude Controller/2(altitude_actual), Display16/1  "z_measured"
  Demux1/2 -> [y_measured]  "y_measured"
  velocity/1 -> Display7/1, Position and Attitude Controller/5(vel)
  Motor Mixer/1(motor2) -> [rpm1_des], Display12/1, Desired rpm Motor 2/1
  Trajectory Generator/3(yaw_des) -> Display5/1, Position and Attitude Controller/3(yaw_des)
  Trajectory Generator/2(vel_des) -> Display4/1, Position and Attitude Controller/2(vel_des)
  Trajectory Generator/1(pos_des) -> Demux/1, Display3/1, Position and Attitude Controller/1(pos_des)
  Time Spot for the Trajectory/1 -> Display1/1, Trajectory Generator/3(timespot)
  Clock1/1 -> Trajectory Generator/1(t)
  Constant/1 -> Display/1, Trajectory Generator/2(homePose)
  Position and Attitude Controller/2(Roll Control) -> Display9/1, Motor Mixer/2(Roll Control)
  Position and Attitude Controller/1(Pitch Control) -> Display8/1, Motor Mixer/1(Pitch Control)
  Position and Attitude Controller/3(Yaw Control) -> Display10/1, Motor Mixer/3(Yaw Control)
  Altitude Controller/1(Throttle) -> Display11/1, Motor Mixer/4(Throttle Control)
  Waypoints/1 -> Display2/1, Trajectory Generator/4(waypoints)
  Transfer Fcn/1 -> Altitude Controller/1(altitude_desired), Display18/1
  Motor Mixer/2(motor1) -> [rpm2_des], Display13/1, Desired rpm Motor 1/1
  Motor Mixer/3(motor4) -> [rpm3_des], Display14/1, Desired rpm Motor 4/1
  Motor Mixer/4(motor3) -> [rpm4_des], Display15/1, Desired rpm Motor 3/1
  connections:
  y/LConn1 -- quadcopterPos_Y/RConn1
  x/LConn1 -- quadcopterPos_X/RConn1
  PS-Simulink Converter/LConn1 -- quadcopterVel_X/RConn1
  z/LConn1 -- quadcopterPos_Z/RConn1
  PS-Simulink Converter1/LConn1 -- quadcopterVel_Y/RConn1
  quadcopterVel_Z/RConn1 -- PS-Simulink Converter2/LConn1
